simulink model "Simulacion_SEPIC_2"  (R2021a)
settings: Solver=ode15s  StartTime=0.0  StopTime=0.1  FixedStep=1e-6  RelTol=1e-7
values from neighbouring files (symbols this model uses):
  Cap1 = (Vout*Duty)/(R_load*Del_Vc1*Fs)    [CONVERSOR_SEPIC.m]
  Cap2 = 10*((Vout*Duty)/(R_load*Del_Vc2*Fs))    [CONVERSOR_SEPIC.m]
  L1 = (Vout*Duty)/(Del_IL1*Fs)    (= 8.13074233678e-05)    [CONVERSOR_SEPIC.m]
  L2 = (Vout*Duty)/(Del_IL2*Fs)    (= 5.60740850812e-05)    [CONVERSOR_SEPIC.m]
  Vout = 12    [CONVERSOR_SEPIC.m]
undefined symbols (not defined in the file or in its folder): den_d, num_d
libraries: spsSeriesRLCBranchLib x8, dspstat3 x5, spsCurrentMeasurementLib x3, spsDiodeLib x1, spsGroundLib x1, spsMosfetLib x1, pid_lib x1, spsPVArrayLib x1, simulink x1, spsSeriesRLCLoadLib x1, spsVoltageMeasurementLib x1, spspowerguiLib x1
settings Model: Creator=SAMP0  LastModifiedBy=SAMP0
settings SolverCC: MaxConsecutiveZCs=10000000

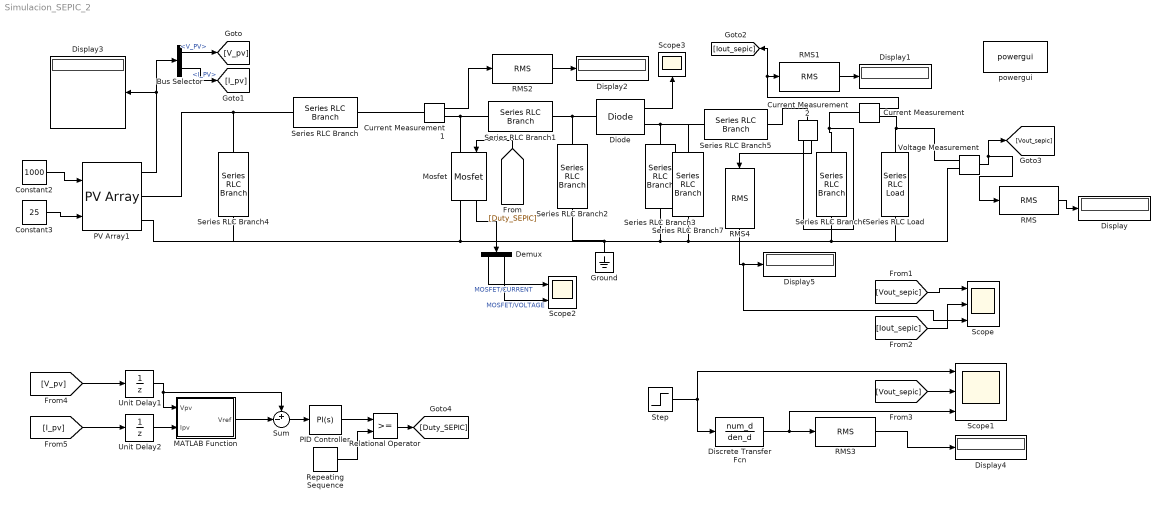
== system Simulacion_SEPIC_2 ==
  Bus Selector : BusSelector  OutputSignals=V_PV,I_PV
  Constant2 : Constant  Value=1000
  Constant3 : Constant  Value=25
  Current Measurement : spsCurrentMeasurementLib/Current Measurement  PhasorSimulation=off  OutputType=Complex  PSBequivalent=0
  Current Measurement1 : spsCurrentMeasurementLib/Current Measurement  PhasorSimulation=off  OutputType=Complex  PSBequivalent=0
  Current Measurement2 : spsCurrentMeasurementLib/Current Measurement  PhasorSimulation=off  OutputType=Complex  PSBequivalent=0
  Demux : Demux  Outputs=2
  Diode : spsDiodeLib/Diode  Ron=0.001  Lon=0  Vf=1  IC=0  UseSnubber=0  Rs=100e6  Cs=250e-9  Measurements=on
  Discrete Transfer Fcn : DiscreteTransferFcn  Numerator=num_d  Denominator=den_d
  Display{,1..5} (6 alike) : Display
  Ground : spsGroundLib/Ground  LConnTagsString=a
  MATLAB Function : MATLAB Function  TreatAsAtomicUnit=on
  Mosfet : spsMosfetLib/Mosfet  Ron=0.1  Lon=0  Rd=0.01  Vfd=0  IC=0  Rs=100e6  Cs=inf  Measurements=on
  PID Controller : pid_lib/PID Controller  Controller=PI  Form=Parallel  TimeDomain=Continuous-time  UseExternalTs=off  SampleTime=-1  IntegratorMethod=Forward Euler  FilterMethod=Forward Euler  ControllerParametersSource=internal  P=0.002  I=0.3  D=0  UseFilter=on  N=100  TunerSelectOption=Transfer Function Based (PID Tuner App)  InitialConditionSource=internal  InitialConditionForIntegrator=0  InitialConditionForFilter=0  DifferentiatorICPrevScaledInput=0  ExternalReset=none  TrackingMode=off  Kt=1  LimitOutput=on  SatLimitsSource=internal  UpperSaturationLimit=0.95  LowerSaturationLimit=0  LinearizeAsGain=on  AntiWindupMode=clamping  Kb=1  POutMin=[]  POutMax=[]  IOutMin=[]  IOutMax=[]  DOutMin=[]  DOutMax=[]  NOutMin=[]  NOutMax=[]  SumOutMin=[]  SumOutMax=[]  SaturationOutMin=[]  SaturationOutMax=[]  PParamMin=[]  PParamMax=[]  IParamMin=[]  IParamMax=[]  DParamMin=[]  DParamMax=[]  NParamMin=[]  NParamMax=[]  KbParamMin=[]  KbParamMax=[]  KtParamMin=[]  KtParamMax=[]  KbOutMin=[]  KbOutMax=[]  KtOutMin=[]  KtOutMax=[]  IntegratorOutMin=[]  IntegratorOutMax=[]  FilterOutMin=[]  FilterOutMax=[]  SumI1OutMin=[]  SumI1OutMax=[]  SumI2OutMin=[]  SumI2OutMax=[]  SumI3OutMin=[]  SumI3OutMax=[]  SumI4OutMin=[]  SumI4OutMax=[]  SumDOutMin=[]  SumDOutMax=[]  DifferentiatorOutMin=[]  DifferentiatorOutMax=[]  FilterDiffOutCoefMin=[]  FilterDiffOutCoefMax=[]  ReciprocalOutMin=[]  ReciprocalOutMax=[]  SumDenOutMin=[]  SumDenOutMax=[]  SumNumOutMin=[]  SumNumOutMax=[]  DivideOutMin=[]  DivideOutMax=[]  UdiffTsProdOutMin=[]  UdiffTsProdOutMax=[]  NTsProdOutMin=[]  NTsProdOutMax=[]  UintegralTsProdOutMin=[]  UintegralTsProdOutMax=[]  UngainTsProdOutMin=[]  UngainTsProdOutMax=[]  IntegratorContinuousStateAttributes=''  IntegratorStateMustResolveToSignalObject=off  IntegratorRTWStateStorageClass=Auto  FilterContinuousStateAttributes=''  FilterStateMustResolveToSignalObject=off  FilterRTWStateStorageClass=Auto  ParallelPVariant=InternalParameters  IdealPVariant=Disabled  IVariant=InternalParameters  DVariant=Disabled  IntegratorVariant=Continuous  SatVariant=Enabled  AWVariant=ContClampingParallel  PCopyVariant=Disabled  TRVariant=Disabled  FdbkBlocksVariant=Forward  IdealPFdbkVariant=Disabled  SatFdbkVariant=Disabled  DerivativeFilterVariant=Disabled  NVariant=Disabled  NCopyVariant=Disabled_SignalSpec  FilterICVariant=Disabled  IntegratorICVariant=InternalICs  ExternalResetVariant=Disabled  TRSumVariant=Passthrough  SumFdbkVariant=Disabled  SumVariant=Sum_PI  TsampFilterVariant=InternalTs  TsampNgainVariant=Passthrough  TsampIntegralVariant=Passthrough  ExternalSaturationOutDataTypeStr=Inherit: Same as second input
  PV Array1 : spsPVArrayLib/PV Array  Npar=1  Nser=1  PlotType=array @ 1000 W/m2 & specified temperatures  S_vec="[ 1000  500  100 ]"  Temp_C_vec="[ 45 25  ]"  ModuleName=User-defined  PlotWhenSelected=off  Pm=87.348  Ncell=72  Voc=21.7  Isc=5.34  Vm=17.4  Im=5.02  beta_Voc_pc=-0.1  alpha_Isc_pc=2.12e-3  beta_Voc=-0.0217  alpha_Isc=0.00011321  IL=5.3604  I0=8.3657e-17  nI=0.30338  Rsh=126.5224  Rs=0.48307  RobustModel=off  RobustCellTemperature=313.3991  BAL=off  Tc=Ts  Tfilter=1e-6
  RMS{,1..4} (5 alike) : dspstat3/RMS  run=off  directionMode=Each column  dimension=1  InputProcessing=Columns as channels (frame based)  reset_popup=None
  Relational Operator : RelationalOperator  OutDataTypeStr=boolean  RndMeth=Simplest
  Repeating Sequence : simulink/Sources/Repeating Sequence  rep_seq_t=[0 1/85e3]  rep_seq_y=[0 1]
  Scope : Scope  NumInputPorts=3
  Scope1 : Scope  NumInputPorts=3
  Scope2 : Scope  NumInputPorts=2
  Scope3 : Scope
  Series RLC Branch : spsSeriesRLCBranchLib/Series RLC Branch  LConnTagsString=__new0  RConnTagsString=__new0  BranchType=L  Resistance=1  Inductance=L1  SetiL0=off  InitialCurrent=0  Capacitance=1e-6  Setx0=off  InitialVoltage=0  Measurements=None
  Series RLC Branch1 : spsSeriesRLCBranchLib/Series RLC Branch  LConnTagsString=__new0  RConnTagsString=__new0  BranchType=C  Resistance=1  Inductance=Cap1  SetiL0=off  InitialCurrent=0  Capacitance=Cap1  Setx0=off  InitialVoltage=0  Measurements=None
  Series RLC Branch2 : spsSeriesRLCBranchLib/Series RLC Branch  LConnTagsString=__new0  RConnTagsString=__new0  BranchType=L  Resistance=1  Inductance=L2  SetiL0=off  InitialCurrent=0  Capacitance=1e-6  Setx0=off  InitialVoltage=0  Measurements=None
  Series RLC Branch3 : spsSeriesRLCBranchLib/Series RLC Branch  LConnTagsString=__new0  RConnTagsString=__new0  BranchType=C  Resistance=1  Inductance=L1  SetiL0=off  InitialCurrent=0  Capacitance=Cap2  Setx0=off  InitialVoltage=0  Measurements=None
  Series RLC Branch4 : spsSeriesRLCBranchLib/Series RLC Branch  LConnTagsString=__new0  RConnTagsString=__new0  BranchType=RC  Resistance=1  Inductance=L1  SetiL0=off  InitialCurrent=0  Capacitance=330e-6  Setx0=off  InitialVoltage=0  Measurements=None
  Series RLC Branch5 : spsSeriesRLCBranchLib/Series RLC Branch  LConnTagsString=__new0  RConnTagsString=__new0  BranchType=L  Resistance=10  Inductance=22e-6  SetiL0=off  InitialCurrent=0  Capacitance=1e-6  Setx0=off  InitialVoltage=0  Measurements=None
  Series RLC Branch6 : spsSeriesRLCBranchLib/Series RLC Branch  LConnTagsString=__new0  RConnTagsString=__new0  BranchType=C  Resistance=1  Inductance=L1  SetiL0=off  InitialCurrent=0  Capacitance=180e-6  Setx0=off  InitialVoltage=0  Measurements=None
  Series RLC Branch7 : spsSeriesRLCBranchLib/Series RLC Branch  LConnTagsString=__new0  RConnTagsString=__new0  BranchType=C  Resistance=1  Inductance=L1  SetiL0=off  InitialCurrent=0  Capacitance=330e-6  Setx0=off  InitialVoltage=0  Measurements=None
  Series RLC Load : spsSeriesRLCLoadLib/Series RLC Load  LConnTagsString=a  RConnTagsString=__new0  NominalVoltage=12  NominalFrequency=0.0000000001  ActivePower=Powr_out  InductivePower=0  CapacitivePower=0  Setx0=off  InitialVoltage=0  SetiL0=off  InitialCurrent=0  Measurements=None  LoadType=constant Z
  Step : Step  Time=0  After=Vout  SampleTime=0
  Sum : Sum  Inputs=+-|
  Unit Delay1 : UnitDelay  SampleTime=-1  HasFrameUpgradeWarning=on
  Unit Delay2 : UnitDelay  SampleTime=-1  HasFrameUpgradeWarning=on
  Voltage Measurement : spsVoltageMeasurementLib/Voltage Measurement  PhasorSimulation=off  OutputType=Complex  PSBequivalent=0
  powergui : spspowerguiLib/powergui  Priority=1  SimulationMode=Discrete  SampleTime=1e-6  frequency=60  Iterations=50  frequencyindice=0  Pbase=100e6  ErrMax=1e-4  UnitsV=kV  UnitsW=MW  buscounter=0  FunctionMessages=off  echomessages=off  EnableUseOfTLC=off  CurrentSourceSwitches=off  DisableSnubberDevices=off  DisableRonSwitches=off  DisableVfSwitches=off  DisplayEquations=off  AutomaticDiscreteSolvers=off  SolverType=Tustin/Backward Euler (TBE)  Interpol=off  ExternalGateDelay=off  methode=off  Ts=100  x0status=blocks  SPID=on  SwTol=0  HookPort=off  NonlinearTolerance=1e-4  nMaxIteration=100  ContinueOnMaxIteration=off  RestoreLinks=warning  ResistiveCurrentMeasurement=off  Frange=[0:2:500]  Ylog=off  Xlog=on  ShowGrid=off  save=off  variable=ZData  structure=0  ZoomFFT=off  StartTime=0.0  cycles=1  DisplayStyle=1  fundamental=60  FreqAxis=off  MaxFrequency=1000  frequencyindicesteady=1  RmsSteady=1  display=off
  wires:
  Current Measurement/1 -> RMS1/1, [Iout_sepic]
  RMS/1 -> Display/1
  RMS1/1 -> Display1/1
  Current Measurement1/1 -> RMS2/1
  RMS2/1 -> Display2/1
  RMS3/1 -> Display4/1
  Demux/1 -> Scope2/1  "MOSFET/CURRENT"
  Demux/2 -> Scope2/2  "MOSFET/VOLTAGE"
  Mosfet/1 -> Demux/1
  Diode/1 -> Scope3/1
  Step/1 -> Discrete Transfer Fcn/1, Scope1/1
  Discrete Transfer Fcn/1 -> Scope1/3, RMS3/1
  Voltage Measurement/1 -> RMS/1, [Vout_sepic]
  Constant3/1 -> PV Array1/2
  Constant2/1 -> PV Array1/1
  PV Array1/1 -> Bus Selector/1, Display3/1
  Bus Selector/1 -> [V_pv]  "<V_PV>"
  Bus Selector/2 -> [I_pv]  "<I_PV>"
  [Vout_sepic] -> Scope/1
  [Iout_sepic] -> Scope/2
  [Vout_sepic] -> Scope1/2
  Unit Delay2/1 -> MATLAB Function/2(Ipv)
  Unit Delay1/1 -> Sum/1, MATLAB Function/1(Vpv)
  MATLAB Function/1(Vref) -> Sum/2
  Sum/1 -> PID Controller/1
  PID Controller/1 -> Relational Operator/1
  Repeating Sequence/1 -> Relational Operator/2
  Relational Operator/1 -> [Duty_SEPIC]
  [Duty_SEPIC] -> Mosfet/1
  [V_pv] -> Unit Delay1/1
  [I_pv] -> Unit Delay2/1
  RMS4/1 -> Scope/3, Display5/1
  Current Measurement2/1 -> RMS4/1
  connections:
  Series RLC Branch1/LConn1 -- Current Measurement1/RConn1 -- Mosfet/LConn1
  Series RLC Branch2/LConn1 -- Diode/LConn1 -- Series RLC Branch1/RConn1
  Current Measurement1/LConn1 -- Series RLC Branch/RConn1
  Series RLC Branch2/RConn1 -- Ground/LConn1 -- Series RLC Load/RConn1 -- Voltage Measurement/LConn2 -- Series RLC Branch6/RConn1 -- Series RLC Branch7/RConn1 -- Series RLC Branch3/RConn1 -- PV Array1/RConn2 -- Series RLC Branch4/RConn1 -- Mosfet/RConn1
  PV Array1/RConn1 -- Series RLC Branch4/LConn1 -- Series RLC Branch/LConn1
  Series RLC Branch3/LConn1 -- Series RLC Branch5/LConn1 -- Series RLC Branch7/LConn1 -- Diode/RConn1
  Voltage Measurement/LConn1 -- Current Measurement/RConn1 -- Series RLC Load/LConn1
  Current Measurement/LConn1 -- Current Measurement2/RConn1 -- Series RLC Branch6/LConn1
  Current Measurement2/LConn1 -- Series RLC Branch5/RConn1

== matlab function Simulacion_SEPIC_2/MATLAB Function ==
  data: Vpv input; Vref output; Ipv input
function Vref = Refgen(Vpv, Ipv)

Vrefmax = 17.4;
Vrefmin = 0;
Vrefinit = 12;

deltaVref = 0.2;

persistent Vold Pold Vrefold;
datatype = 'double';

if isempty(Vold)
    Vold = 0;
    Pold = 0;
    Vrefold = Vrefinit;
end

Ppv = Vpv * Ipv;
dV = Vpv - Vold;
dP = Ppv - Pold;

if dP ~= 0
   if dP < 0
       if dV < 0 
           Vref = Vrefold + deltaVref;
       else
           Vref = Vrefold - deltaVref;
       end
   else
       if dV < 0 
           Vref = Vrefold - deltaVref;
       else
           Vref = Vrefold + deltaVref;
       end
   end
else
    Vref = Vrefold;
end

if Vref >= Vrefmax | Vref <= Vrefmin
    Vref = Vrefold;
end

Vrefold = Vref;
Vold = Vpv;
Pold = Ppv;
